simulink model "SCLAING_TRAINING_39"  (R2021a)
settings: Solver=ode23tb  StartTime=0.0  StopTime=27  MaxStep=1/60  RelTol=1e-2  AbsTol=1e-1  EnableMultiTasking=on
PreLoadFcn:
  | NE39bus_data;
  | PSSMODEL=1;
  | LPSS=0;
  | WAPSS=0;
  | WAPSS2=0;
undefined symbols (not defined in the file): AVR_Data, D1, Delta, line, mac_con, MB, Ns, p0, Pn, s
libraries: spsThreePhaseVIMeasurementLib x40, spsThreePhasePISectionLineLib x34, simulink x20, spsGenericPowerSystemStabilizerLib x20, spsThreePhaseTransformerTwoWindingsLib x12, spsSynchronousMachinepuStandardLib x10, spsExcitationSystemLib x10, spsMultiBandPowerSystemStabilizerLib x10, spsSteamTurbineandGovernorLib x10, slpidlib x10, spsLoadFlowBusLib x9, spsThreePhaseDynamicLoadLib x9
(part 4 of 4)

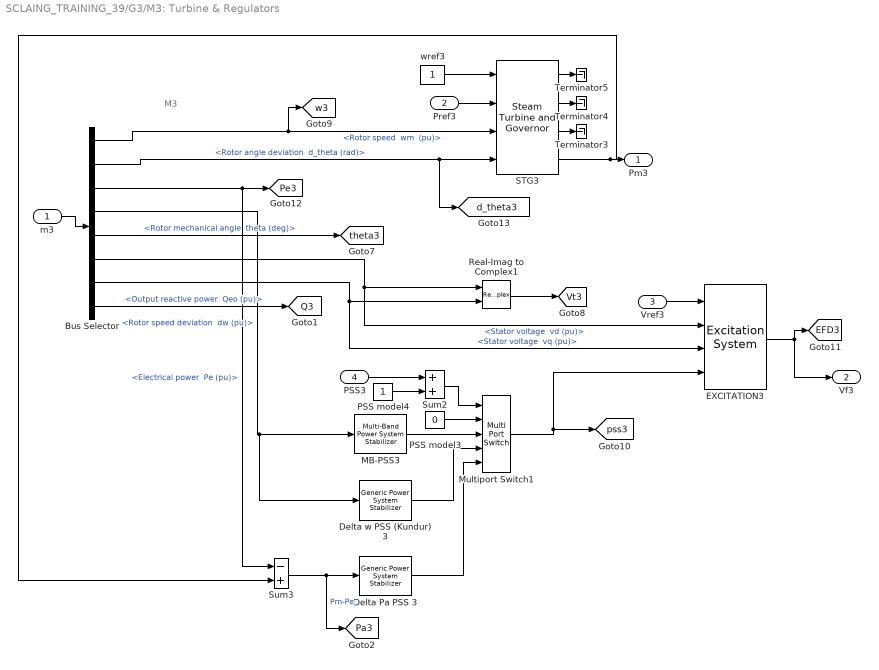
== system SCLAING_TRAINING_39/G3/M3: Turbine & Regulators ==
  note: M3
  m3 : Inport
  Pref3 : Inport  Port=2
  Vref3 : Inport  Port=3
  PSS3 : Inport  Port=4
  Bus Selector : BusSelector  OutputSignals="Mechanical.Rotor speed  wm  (pu),Mechanical.Rotor angle deviation  d_theta (rad),Mechanical.Electrical power  Pe (pu),Mechanical.Rotor speed deviation  dw (pu),Mechanical.Rotor mechanical angle  theta (deg),dq0 components.Stator voltage  vd (pu),dq0 components.Stator voltage  vq (pu),Output reactive power  Qeo (pu)"
  Delta Pa PSS 3 : spsGenericPowerSystemStabilizerLib/Generic Power System Stabilizer  Tsensor=15e-3  K=2.5*1.25  Twashout=1  Tleadlag1=[60e-3 1]  Tleadlag2=[0 0]  VSlimits=[-0.15 0.15]  Vinit=0  Plot_On=off  MagdB_On=on  FreqRange=logspace(-2,2,500)
      settings: SourceProductBaseCode=PS
  Delta w PSS (Kundur) 3 : spsGenericPowerSystemStabilizerLib/Generic Power System Stabilizer  Tsensor=15e-3  K=30  Twashout=10  Tleadlag1=[50e-3 20e-3]  Tleadlag2=[3 5.4]  VSlimits=[-0.15 0.15]  Vinit=0  Plot_On=off  MagdB_On=on  FreqRange=logspace(-2,2,500)
      settings: SourceProductBaseCode=PS
  EXCITATION3 : spsExcitationSystemLib/Excitation System  tr=AVR_Data(3,1)  reg=[ AVR_Data(3,2:3) ]  exc=[ 1, 0 ]  tgr=[ AVR_Data(3,4:5)]  damp=[ 0, 0 ]  sat=[ 0, 0 ]  lim="[ AVR_Data(3,7:8)  0 ]"  v0=[1,2.25944]
      settings: SourceProductBaseCode=PS
  MB-PSS3 : spsMultiBandPowerSystemStabilizerLib/Multi-Band Power System Stabilizer  OperationMode=Simplified settings  Kg=MB(1)  GL=[MB(2) MB(3)]  GI=[MB(4) MB(5)]  GH=[MB(6) MB(7)]  GLd=[66 66 9.4]  TcLF=[1.667 2 0 0 0 0 2 2.4 0 0 0 0 1 1]  GId=[66 66 47.6]  TcIF=[1 1 0.25 0.3 0 0 1 1 0.3 0.36 0 0 0 0]  GHd=[66 66 233]  TcHF="[0.01 0.012 0 0 0 0  0.012 0.0144 0 0 0 0 1 1]"  LIM=[.075 .15 .15 .15]  Plot_On=off  MagdB_On=off  FreqRange=logspace(-2,2,500)
      settings: SourceProductBaseCode=PS
  Multiport Switch1 : MultiPortSwitch  Inputs=4  InputSameDT=on
  PSS model3 : Constant  Value=0
  PSS model4 : Constant
  Real-Imag to Complex1 : RealImagToComplex
  STG3 : spsSteamTurbineandGovernorLib/Steam Turbine and Governor  gentype=Tandem-compound (single mass)  reg1="[ 1  0.05    0 ]"  reg2="[ 0.001  0.15 ]"  reg3="[ -0.1  0.1  0  4.496 ]"  N=Ns  turb1="[ 0  10   3.3   0.5   ]"  turb2="[   0   0.36    0.36   0.28   ]"  HA="[ 0.046  1.430  1.465   0.192 ]"  KA="[ 90.44  53.88  64.59   62.94  ]"  DA="[ 0.0115  0.3575  0.3663   0.0137  ]"  ini1=0.65  ini2=[0.779316,-31.4247]
      settings: SourceProductBaseCode=PS
  Sum2 : Sum  InputSameDT=on  SaturateOnIntegerOverflow=on  OutDataTypeStr=Inherit: Same as first input
  Sum3 : Sum  Inputs=-+  InputSameDT=on  SaturateOnIntegerOverflow=on  OutDataTypeStr=Inherit: Same as first input
  Terminator3 : Terminator
  Terminator4 : Terminator
  Terminator5 : Terminator
  wref3 : Constant
  Pm3 : Outport  InitialOutput=0
  Vf3 : Outport  Port=2  InitialOutput=0
  tag scope: EFD3=global, Pa3=global, Pe3=global, Q3=global, Vt3=global, d_theta3=global, pss3=global, theta3=global, w3=global
  wires:
  Bus Selector/7 -> EXCITATION3/3, Real-Imag to Complex1/2  "<Stator voltage  vq (pu)>"
  wref3/1 -> STG3/1
  Pref3/1 -> STG3/2
  m3/1 -> Bus Selector/1
  Vref3/1 -> EXCITATION3/1
  EXCITATION3/1 -> Vf3/1, [EFD3]
  Real-Imag to Complex1/1 -> [Vt3]
  Bus Selector/5 -> [theta3]  "<Rotor mechanical angle  theta (deg)>"
  Bus Selector/6 -> EXCITATION3/2, Real-Imag to Complex1/1  "<Stator voltage  vd (pu)>"
  STG3/3 -> Terminator3/1
  STG3/4 -> Sum3/2, Pm3/1
  STG3/2 -> Terminator4/1
  STG3/1 -> Terminator5/1
  Bus Selector/1 -> [w3], STG3/3  "<Rotor speed  wm  (pu)>"
  Bus Selector/2 -> STG3/4, [d_theta3]  "<Rotor angle deviation  d_theta (rad)>"
  Bus Selector/3 -> Sum3/1, [Pe3]  "<Electrical power  Pe (pu)>"
  Bus Selector/4 -> Delta w PSS (Kundur) 3/1, MB-PSS3/1  "<Rotor speed deviation  dw (pu)>"
  Bus Selector/8 -> [Q3]  "<Output reactive power  Qeo (pu)>"
  Sum3/1 -> [Pa3], Delta Pa PSS 3/1  "Pm-Pe"
  Sum2/1 -> Multiport Switch1/1
  PSS model4/1 -> Sum2/2
  Delta Pa PSS 3/1 -> Multiport Switch1/5
  Delta w PSS (Kundur) 3/1 -> Multiport Switch1/4
  MB-PSS3/1 -> Multiport Switch1/3
  PSS model3/1 -> Multiport Switch1/2
  Multiport Switch1/1 -> EXCITATION3/4, [pss3]
  PSS3/1 -> Sum2/1

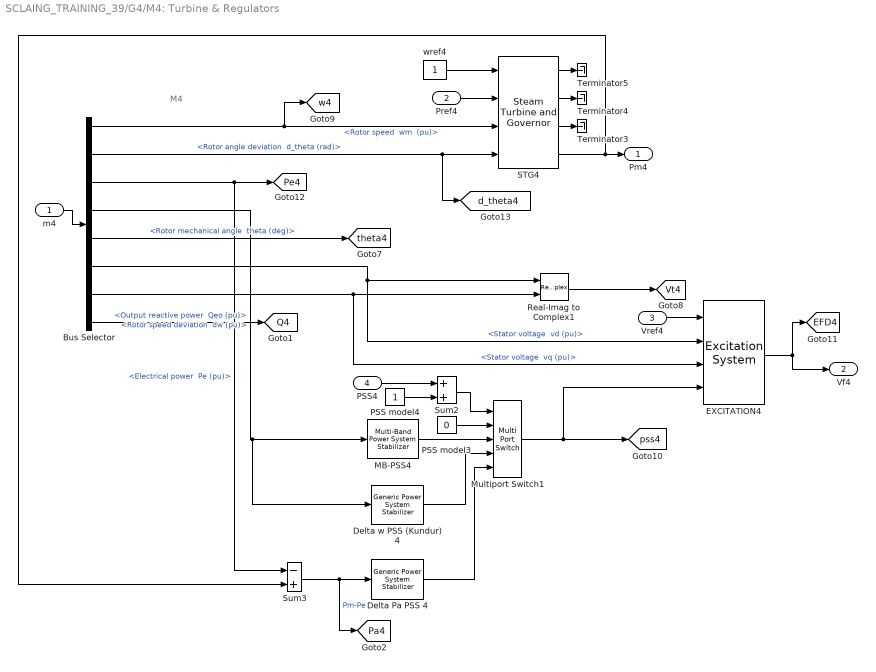
== system SCLAING_TRAINING_39/G4/M4: Turbine & Regulators ==
  note: M4
  m4 : Inport
  Pref4 : Inport  Port=2
  Vref4 : Inport  Port=3
  PSS4 : Inport  Port=4
  Bus Selector : BusSelector  OutputSignals="Mechanical.Rotor speed  wm  (pu),Mechanical.Rotor angle deviation  d_theta (rad),Mechanical.Electrical power  Pe (pu),Mechanical.Rotor speed deviation  dw (pu),Mechanical.Rotor mechanical angle  theta (deg),dq0 components.Stator voltage  vd (pu),dq0 components.Stator voltage  vq (pu),Output reactive power  Qeo (pu)"
  Delta Pa PSS 4 : spsGenericPowerSystemStabilizerLib/Generic Power System Stabilizer  Tsensor=15e-3  K=2.5*1.25  Twashout=1  Tleadlag1=[60e-3 1]  Tleadlag2=[0 0]  VSlimits=[-0.15 0.15]  Vinit=0  Plot_On=off  MagdB_On=on  FreqRange=logspace(-2,2,500)
      settings: SourceProductBaseCode=PS
  Delta w PSS (Kundur) 4 : spsGenericPowerSystemStabilizerLib/Generic Power System Stabilizer  Tsensor=15e-3  K=30  Twashout=10  Tleadlag1=[50e-3 20e-3]  Tleadlag2=[3 5.4]  VSlimits=[-0.15 0.15]  Vinit=0  Plot_On=off  MagdB_On=on  FreqRange=logspace(-2,2,500)
      settings: SourceProductBaseCode=PS
  EXCITATION4 : spsExcitationSystemLib/Excitation System  tr=AVR_Data(1)  reg=[ AVR_Data(4,2:3) ]  exc=[ 1, 0 ]  tgr=[ AVR_Data(4,4:5)]  damp=[ 0, 0 ]  sat=[ 0, 0 ]  lim="[ AVR_Data(4,7:8)  0 ]"  v0=[1,2.14879]
      settings: SourceProductBaseCode=PS
  MB-PSS4 : spsMultiBandPowerSystemStabilizerLib/Multi-Band Power System Stabilizer  OperationMode=Simplified settings  Kg=MB(1)  GL=[MB(2) MB(3)]  GI=[MB(4) MB(5)]  GH=[MB(6) MB(7)]  GLd=[66 66 9.4]  TcLF=[1.667 2 0 0 0 0 2 2.4 0 0 0 0 1 1]  GId=[66 66 47.6]  TcIF=[1 1 0.25 0.3 0 0 1 1 0.3 0.36 0 0 0 0]  GHd=[66 66 233]  TcHF="[0.01 0.012 0 0 0 0  0.012 0.0144 0 0 0 0 1 1]"  LIM=[.075 .15 .15 .15]  Plot_On=off  MagdB_On=off  FreqRange=logspace(-2,2,500)
      settings: SourceProductBaseCode=PS
  Multiport Switch1 : MultiPortSwitch  Inputs=4  InputSameDT=on
  PSS model3 : Constant  Value=0
  PSS model4 : Constant
  Real-Imag to Complex1 : RealImagToComplex
  STG4 : spsSteamTurbineandGovernorLib/Steam Turbine and Governor  gentype=Tandem-compound (single mass)  reg1="[ 1  0.05    0 ]"  reg2="[ 0.001  0.15 ]"  reg3="[ -0.1  0.1  0  4.496 ]"  N=Ns  turb1="[ 0  10   3.3   0.5   ]"  turb2="[   0   0.36    0.36   0.28   ]"  HA="[ 0.046  1.430  1.465   0.192 ]"  KA="[ 90.44  53.88  64.59   62.94  ]"  DA="[ 0.0115  0.3575  0.3663   0.0137  ]"  ini1=0.632  ini2=[0.779316,-31.4247]
      settings: SourceProductBaseCode=PS
  Sum2 : Sum  InputSameDT=on  SaturateOnIntegerOverflow=on  OutDataTypeStr=Inherit: Same as first input
  Sum3 : Sum  Inputs=-+  InputSameDT=on  SaturateOnIntegerOverflow=on  OutDataTypeStr=Inherit: Same as first input
  Terminator3 : Terminator
  Terminator4 : Terminator
  Terminator5 : Terminator
  wref4 : Constant
  Pm4 : Outport  InitialOutput=0
  Vf4 : Outport  Port=2  InitialOutput=0
  tag scope: EFD4=global, Pa4=global, Pe4=global, Q4=global, Vt4=global, d_theta4=global, pss4=global, theta4=global, w4=global
  wires:
  Bus Selector/7 -> EXCITATION4/3, Real-Imag to Complex1/2  "<Stator voltage  vq (pu)>"
  wref4/1 -> STG4/1
  Pref4/1 -> STG4/2
  m4/1 -> Bus Selector/1
  Vref4/1 -> EXCITATION4/1
  EXCITATION4/1 -> Vf4/1, [EFD4]
  Real-Imag to Complex1/1 -> [Vt4]
  Bus Selector/5 -> [theta4]  "<Rotor mechanical angle  theta (deg)>"
  Bus Selector/6 -> EXCITATION4/2, Real-Imag to Complex1/1  "<Stator voltage  vd (pu)>"
  STG4/3 -> Terminator3/1
  STG4/4 -> Sum3/2, Pm4/1
  STG4/2 -> Terminator4/1
  STG4/1 -> Terminator5/1
  Bus Selector/1 -> [w4], STG4/3  "<Rotor speed  wm  (pu)>"
  Bus Selector/2 -> [d_theta4], STG4/4  "<Rotor angle deviation  d_theta (rad)>"
  Bus Selector/3 -> Sum3/1, [Pe4]  "<Electrical power  Pe (pu)>"
  Bus Selector/4 -> Delta w PSS (Kundur) 4/1, MB-PSS4/1  "<Rotor speed deviation  dw (pu)>"
  Bus Selector/8 -> [Q4]  "<Output reactive power  Qeo (pu)>"
  Sum3/1 -> [Pa4], Delta Pa PSS 4/1  "Pm-Pe"
  Sum2/1 -> Multiport Switch1/1
  PSS model4/1 -> Sum2/2
  Delta Pa PSS 4/1 -> Multiport Switch1/5
  Delta w PSS (Kundur) 4/1 -> Multiport Switch1/4
  MB-PSS4/1 -> Multiport Switch1/3
  PSS model3/1 -> Multiport Switch1/2
  Multiport Switch1/1 -> [pss4], EXCITATION4/4
  PSS4/1 -> Sum2/1

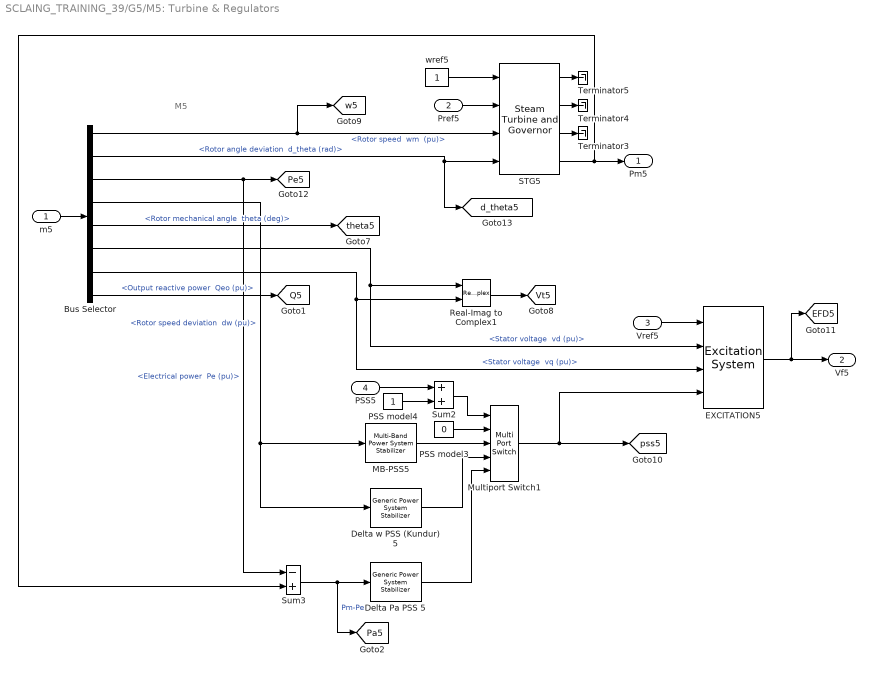
== system SCLAING_TRAINING_39/G5/M5: Turbine & Regulators ==
  note: M5
  m5 : Inport
  Pref5 : Inport  Port=2
  Vref5 : Inport  Port=3
  PSS5 : Inport  Port=4
  Bus Selector : BusSelector  OutputSignals="Mechanical.Rotor speed  wm  (pu),Mechanical.Rotor angle deviation  d_theta (rad),Mechanical.Electrical power  Pe (pu),Mechanical.Rotor speed deviation  dw (pu),Mechanical.Rotor mechanical angle  theta (deg),dq0 components.Stator voltage  vd (pu),dq0 components.Stator voltage  vq (pu),Output reactive power  Qeo (pu)"
  Delta Pa PSS 5 : spsGenericPowerSystemStabilizerLib/Generic Power System Stabilizer  Tsensor=15e-3  K=2.5*1.25  Twashout=1  Tleadlag1=[60e-3 1]  Tleadlag2=[0 0]  VSlimits=[-0.15 0.15]  Vinit=0  Plot_On=off  MagdB_On=on  FreqRange=logspace(-2,2,500)
      settings: SourceProductBaseCode=PS
  Delta w PSS (Kundur) 5 : spsGenericPowerSystemStabilizerLib/Generic Power System Stabilizer  Tsensor=15e-3  K=30  Twashout=10  Tleadlag1=[50e-3 20e-3]  Tleadlag2=[3 5.4]  VSlimits=[-0.15 0.15]  Vinit=0  Plot_On=off  MagdB_On=on  FreqRange=logspace(-2,2,500)
      settings: SourceProductBaseCode=PS
  EXCITATION5 : spsExcitationSystemLib/Excitation System  tr=AVR_Data(5,1)  reg=[ AVR_Data(5,2:3) ]  exc=[ 1, 0 ]  tgr=[ AVR_Data(5,4:5)]  damp=[ 0, 0 ]  sat=[ 0, 0 ]  lim="[ AVR_Data(5,7:8)  0 ]"  v0=[1,3.89055]
      settings: SourceProductBaseCode=PS
  MB-PSS5 : spsMultiBandPowerSystemStabilizerLib/Multi-Band Power System Stabilizer  OperationMode=Simplified settings  Kg=MB(1)  GL=[MB(2) MB(3)]  GI=[MB(4) MB(5)]  GH=[MB(6) MB(7)]  GLd=[66 66 9.4]  TcLF=[1.667 2 0 0 0 0 2 2.4 0 0 0 0 1 1]  GId=[66 66 47.6]  TcIF=[1 1 0.25 0.3 0 0 1 1 0.3 0.36 0 0 0 0]  GHd=[66 66 233]  TcHF="[0.01 0.012 0 0 0 0  0.012 0.0144 0 0 0 0 1 1]"  LIM=[.075 .15 .15 .15]  Plot_On=off  MagdB_On=off  FreqRange=logspace(-2,2,500)
      settings: SourceProductBaseCode=PS
  Multiport Switch1 : MultiPortSwitch  Inputs=4  InputSameDT=on
  PSS model3 : Constant  Value=0
  PSS model4 : Constant
  Real-Imag to Complex1 : RealImagToComplex
  STG5 : spsSteamTurbineandGovernorLib/Steam Turbine and Governor  gentype=Tandem-compound (single mass)  reg1="[ 1  0.05    0 ]"  reg2="[ 0.001  0.15 ]"  reg3="[ -0.1  0.1  0  4.496 ]"  N=Ns  turb1="[ 0  10   3.3   0.5   ]"  turb2="[   0   0.36    0.36   0.28   ]"  HA="[ 0.046  1.430  1.465   0.192 ]"  KA="[ 90.44  53.88  64.59   62.94  ]"  DA="[ 0.0115  0.3575  0.3663   0.0137  ]"  ini1=0.508  ini2=[0.779316,-31.4247]
      settings: SourceProductBaseCode=PS
  Sum2 : Sum  InputSameDT=on  SaturateOnIntegerOverflow=on  OutDataTypeStr=Inherit: Same as first input
  Sum3 : Sum  Inputs=-+  InputSameDT=on  SaturateOnIntegerOverflow=on  OutDataTypeStr=Inherit: Same as first input
  Terminator3 : Terminator
  Terminator4 : Terminator
  Terminator5 : Terminator
  wref5 : Constant
  Pm5 : Outport  InitialOutput=0
  Vf5 : Outport  Port=2  InitialOutput=0
  tag scope: EFD5=global, Pa5=global, Pe5=global, Q5=global, Vt5=global, d_theta5=global, pss5=global, theta5=global, w5=global
  wires:
  Bus Selector/7 -> EXCITATION5/3, Real-Imag to Complex1/2  "<Stator voltage  vq (pu)>"
  wref5/1 -> STG5/1
  Pref5/1 -> STG5/2
  m5/1 -> Bus Selector/1
  Vref5/1 -> EXCITATION5/1
  EXCITATION5/1 -> Vf5/1, [EFD5]
  Real-Imag to Complex1/1 -> [Vt5]
  Bus Selector/5 -> [theta5]  "<Rotor mechanical angle  theta (deg)>"
  Bus Selector/6 -> EXCITATION5/2, Real-Imag to Complex1/1  "<Stator voltage  vd (pu)>"
  STG5/3 -> Terminator3/1
  STG5/4 -> Sum3/2, Pm5/1
  STG5/2 -> Terminator4/1
  STG5/1 -> Terminator5/1
  Bus Selector/1 -> [w5], STG5/3  "<Rotor speed  wm  (pu)>"
  Bus Selector/2 -> [d_theta5], STG5/4  "<Rotor angle deviation  d_theta (rad)>"
  Bus Selector/3 -> Sum3/1, [Pe5]  "<Electrical power  Pe (pu)>"
  Bus Selector/4 -> Delta w PSS (Kundur) 5/1, MB-PSS5/1  "<Rotor speed deviation  dw (pu)>"
  Bus Selector/8 -> [Q5]  "<Output reactive power  Qeo (pu)>"
  Sum3/1 -> [Pa5], Delta Pa PSS 5/1  "Pm-Pe"
  Sum2/1 -> Multiport Switch1/1
  PSS model4/1 -> Sum2/2
  Delta Pa PSS 5/1 -> Multiport Switch1/5
  Delta w PSS (Kundur) 5/1 -> Multiport Switch1/4
  MB-PSS5/1 -> Multiport Switch1/3
  PSS model3/1 -> Multiport Switch1/2
  Multiport Switch1/1 -> [pss5], EXCITATION5/4
  PSS5/1 -> Sum2/1

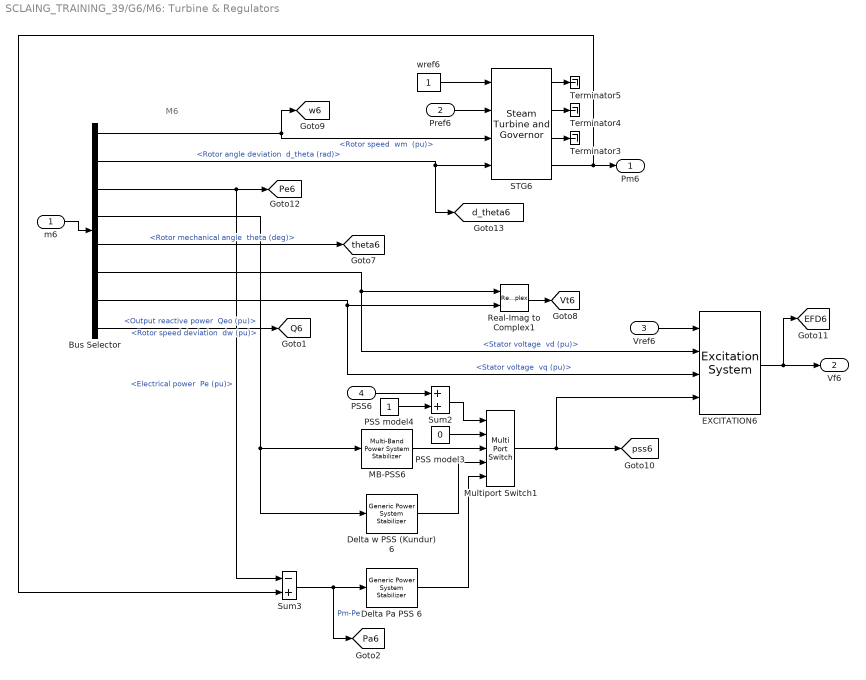
== system SCLAING_TRAINING_39/G6/M6: Turbine & Regulators ==
  note: M6
  m6 : Inport
  Pref6 : Inport  Port=2
  Vref6 : Inport  Port=3
  PSS6 : Inport  Port=4
  Bus Selector : BusSelector  OutputSignals="Mechanical.Rotor speed  wm  (pu),Mechanical.Rotor angle deviation  d_theta (rad),Mechanical.Electrical power  Pe (pu),Mechanical.Rotor speed deviation  dw (pu),Mechanical.Rotor mechanical angle  theta (deg),dq0 components.Stator voltage  vd (pu),dq0 components.Stator voltage  vq (pu),Output reactive power  Qeo (pu)"
  Delta Pa PSS 6 : spsGenericPowerSystemStabilizerLib/Generic Power System Stabilizer  Tsensor=15e-3  K=2.5*1.25  Twashout=1  Tleadlag1=[60e-3 1]  Tleadlag2=[0 0]  VSlimits=[-0.15 0.15]  Vinit=0  Plot_On=off  MagdB_On=on  FreqRange=logspace(-2,2,500)
      settings: SourceProductBaseCode=PS
  Delta w PSS (Kundur) 6 : spsGenericPowerSystemStabilizerLib/Generic Power System Stabilizer  Tsensor=15e-3  K=30  Twashout=10  Tleadlag1=[50e-3 20e-3]  Tleadlag2=[3 5.4]  VSlimits=[-0.15 0.15]  Vinit=0  Plot_On=off  MagdB_On=on  FreqRange=logspace(-2,2,500)
      settings: SourceProductBaseCode=PS
  EXCITATION6 : spsExcitationSystemLib/Excitation System  tr=AVR_Data(6,1)  reg=[ AVR_Data(6,2:3) ]  exc=[ 1, 0 ]  tgr=[ AVR_Data(6,4:5)]  damp=[ 0, 0 ]  sat=[ 0, 0 ]  lim="[ AVR_Data(6,7:8)  0 ]"  v0=[1,2.21937]
      settings: SourceProductBaseCode=PS
  MB-PSS6 : spsMultiBandPowerSystemStabilizerLib/Multi-Band Power System Stabilizer  OperationMode=Simplified settings  Kg=MB(1)  GL=[MB(2) MB(3)]  GI=[MB(4) MB(5)]  GH=[MB(6) MB(7)]  GLd=[66 66 9.4]  TcLF=[1.667 2 0 0 0 0 2 2.4 0 0 0 0 1 1]  GId=[66 66 47.6]  TcIF=[1 1 0.25 0.3 0 0 1 1 0.3 0.36 0 0 0 0]  GHd=[66 66 233]  TcHF="[0.01 0.012 0 0 0 0  0.012 0.0144 0 0 0 0 1 1]"  LIM=[.075 .15 .15 .15]  Plot_On=off  MagdB_On=off  FreqRange=logspace(-2,2,500)
      settings: SourceProductBaseCode=PS
  Multiport Switch1 : MultiPortSwitch  Inputs=4  InputSameDT=on
  PSS model3 : Constant  Value=0
  PSS model4 : Constant
  Real-Imag to Complex1 : RealImagToComplex
  STG6 : spsSteamTurbineandGovernorLib/Steam Turbine and Governor  gentype=Tandem-compound (single mass)  reg1="[ 1  0.05    0 ]"  reg2="[ 0.001  0.15 ]"  reg3="[ -0.1  0.1  0  4.496 ]"  N=Ns  turb1="[ 0  10   3.3   0.5   ]"  turb2="[   0   0.36    0.36   0.28   ]"  HA="[ 0.046  1.430  1.465   0.192 ]"  KA="[ 90.44  53.88  64.59   62.94  ]"  DA="[ 0.0115  0.3575  0.3663   0.0137  ]"  ini1=0.65  ini2=[0.779316,-31.4247]
      settings: SourceProductBaseCode=PS
  Sum2 : Sum  InputSameDT=on  SaturateOnIntegerOverflow=on  OutDataTypeStr=Inherit: Same as first input
  Sum3 : Sum  Inputs=-+  InputSameDT=on  SaturateOnIntegerOverflow=on  OutDataTypeStr=Inherit: Same as first input
  Terminator3 : Terminator
  Terminator4 : Terminator
  Terminator5 : Terminator
  wref6 : Constant
  Pm6 : Outport  InitialOutput=0
  Vf6 : Outport  Port=2  InitialOutput=0
  tag scope: EFD6=global, Pa6=global, Pe6=global, Q6=global, Vt6=global, d_theta6=global, pss6=global, theta6=global, w6=global
  wires:
  Bus Selector/7 -> EXCITATION6/3, Real-Imag to Complex1/2  "<Stator voltage  vq (pu)>"
  wref6/1 -> STG6/1
  Pref6/1 -> STG6/2
  m6/1 -> Bus Selector/1
  Vref6/1 -> EXCITATION6/1
  EXCITATION6/1 -> Vf6/1, [EFD6]
  Real-Imag to Complex1/1 -> [Vt6]
  Bus Selector/5 -> [theta6]  "<Rotor mechanical angle  theta (deg)>"
  Bus Selector/6 -> EXCITATION6/2, Real-Imag to Complex1/1  "<Stator voltage  vd (pu)>"
  STG6/3 -> Terminator3/1
  STG6/4 -> Sum3/2, Pm6/1
  STG6/2 -> Terminator4/1
  STG6/1 -> Terminator5/1
  Bus Selector/1 -> STG6/3, [w6]  "<Rotor speed  wm  (pu)>"
  Bus Selector/2 -> [d_theta6], STG6/4  "<Rotor angle deviation  d_theta (rad)>"
  Bus Selector/3 -> Sum3/1, [Pe6]  "<Electrical power  Pe (pu)>"
  Bus Selector/4 -> Delta w PSS (Kundur) 6/1, MB-PSS6/1  "<Rotor speed deviation  dw (pu)>"
  Bus Selector/8 -> [Q6]  "<Output reactive power  Qeo (pu)>"
  Sum3/1 -> [Pa6], Delta Pa PSS 6/1  "Pm-Pe"
  Sum2/1 -> Multiport Switch1/1
  PSS model4/1 -> Sum2/2
  Delta Pa PSS 6/1 -> Multiport Switch1/5
  Delta w PSS (Kundur) 6/1 -> Multiport Switch1/4
  MB-PSS6/1 -> Multiport Switch1/3
  PSS model3/1 -> Multiport Switch1/2
  Multiport Switch1/1 -> [pss6], EXCITATION6/4
  PSS6/1 -> Sum2/1

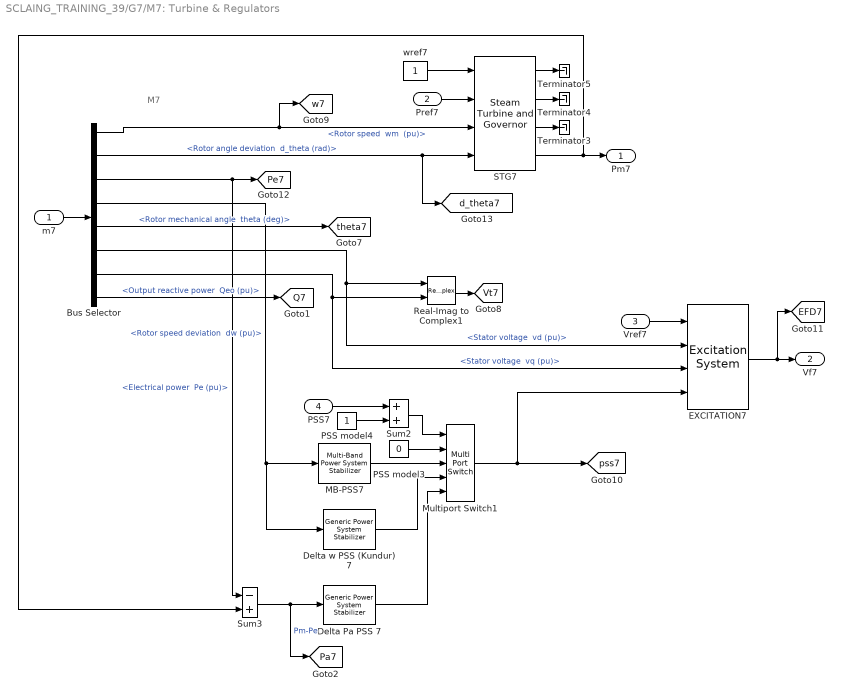
== system SCLAING_TRAINING_39/G7/M7: Turbine & Regulators ==
  note: M7
  m7 : Inport
  Pref7 : Inport  Port=2
  Vref7 : Inport  Port=3
  PSS7 : Inport  Port=4
  Bus Selector : BusSelector  OutputSignals="Mechanical.Rotor speed  wm  (pu),Mechanical.Rotor angle deviation  d_theta (rad),Mechanical.Electrical power  Pe (pu),Mechanical.Rotor speed deviation  dw (pu),Mechanical.Rotor mechanical angle  theta (deg),dq0 components.Stator voltage  vd (pu),dq0 components.Stator voltage  vq (pu),Output reactive power  Qeo (pu)"
  Delta Pa PSS 7 : spsGenericPowerSystemStabilizerLib/Generic Power System Stabilizer  Tsensor=15e-3  K=2.5*1.25  Twashout=1  Tleadlag1=[60e-3 1]  Tleadlag2=[0 0]  VSlimits=[-0.15 0.15]  Vinit=0  Plot_On=off  MagdB_On=on  FreqRange=logspace(-2,2,500)
      settings: SourceProductBaseCode=PS
  Delta w PSS (Kundur) 7 : spsGenericPowerSystemStabilizerLib/Generic Power System Stabilizer  Tsensor=15e-3  K=30  Twashout=10  Tleadlag1=[50e-3 20e-3]  Tleadlag2=[3 5.4]  VSlimits=[-0.15 0.15]  Vinit=0  Plot_On=off  MagdB_On=on  FreqRange=logspace(-2,2,500)
      settings: SourceProductBaseCode=PS
  EXCITATION7 : spsExcitationSystemLib/Excitation System  tr=AVR_Data(7,1)  reg=[ AVR_Data(7,2:3) ]  exc=[ 1, 0 ]  tgr=[ AVR_Data(7,4:5)]  damp=[ 0, 0 ]  sat=[ 0, 0 ]  lim="[ AVR_Data(7,7:8)  0 ]"  v0=[1,2.15543]
      settings: SourceProductBaseCode=PS
  MB-PSS7 : spsMultiBandPowerSystemStabilizerLib/Multi-Band Power System Stabilizer  OperationMode=Simplified settings  Kg=MB(1)  GL=[MB(2) MB(3)]  GI=[MB(4) MB(5)]  GH=[MB(6) MB(7)]  GLd=[66 66 9.4]  TcLF=[1.667 2 0 0 0 0 2 2.4 0 0 0 0 1 1]  GId=[66 66 47.6]  TcIF=[1 1 0.25 0.3 0 0 1 1 0.3 0.36 0 0 0 0]  GHd=[66 66 233]  TcHF="[0.01 0.012 0 0 0 0  0.012 0.0144 0 0 0 0 1 1]"  LIM=[.075 .15 .15 .15]  Plot_On=off  MagdB_On=off  FreqRange=logspace(-2,2,500)
      settings: SourceProductBaseCode=PS
  Multiport Switch1 : MultiPortSwitch  Inputs=4  InputSameDT=on
  PSS model3 : Constant  Value=0
  PSS model4 : Constant
  Real-Imag to Complex1 : RealImagToComplex
  STG7 : spsSteamTurbineandGovernorLib/Steam Turbine and Governor  gentype=Tandem-compound (single mass)  reg1="[ 1  0.05    0 ]"  reg2="[ 0.001  0.15 ]"  reg3="[ -0.1  0.1  0  4.496 ]"  N=Ns  turb1="[ 0  10   3.3   0.5   ]"  turb2="[   0   0.36    0.36   0.28   ]"  HA="[ 0.046  1.430  1.465   0.192 ]"  KA="[ 90.44  53.88  64.59   62.94  ]"  DA="[ 0.0115  0.3575  0.3663   0.0137  ]"  ini1=0.56  ini2=[0.779316,-31.4247]
      settings: SourceProductBaseCode=PS
  Sum2 : Sum  InputSameDT=on  SaturateOnIntegerOverflow=on  OutDataTypeStr=Inherit: Same as first input
  Sum3 : Sum  Inputs=-+  InputSameDT=on  SaturateOnIntegerOverflow=on  OutDataTypeStr=Inherit: Same as first input
  Terminator3 : Terminator
  Terminator4 : Terminator
  Terminator5 : Terminator
  wref7 : Constant
  Pm7 : Outport  InitialOutput=0
  Vf7 : Outport  Port=2  InitialOutput=0
  tag scope: EFD7=global, Pa7=global, Pe7=global, Q7=global, Vt7=global, d_theta7=global, pss7=global, theta7=global, w7=global
  wires:
  Bus Selector/7 -> EXCITATION7/3, Real-Imag to Complex1/2  "<Stator voltage  vq (pu)>"
  wref7/1 -> STG7/1
  Pref7/1 -> STG7/2
  m7/1 -> Bus Selector/1
  Vref7/1 -> EXCITATION7/1
  EXCITATION7/1 -> Vf7/1, [EFD7]
  Real-Imag to Complex1/1 -> [Vt7]
  Bus Selector/5 -> [theta7]  "<Rotor mechanical angle  theta (deg)>"
  Bus Selector/6 -> EXCITATION7/2, Real-Imag to Complex1/1  "<Stator voltage  vd (pu)>"
  STG7/3 -> Terminator3/1
  STG7/4 -> Sum3/2, Pm7/1
  STG7/2 -> Terminator4/1
  STG7/1 -> Terminator5/1
  Bus Selector/1 -> [w7], STG7/3  "<Rotor speed  wm  (pu)>"
  Bus Selector/2 -> STG7/4, [d_theta7]  "<Rotor angle deviation  d_theta (rad)>"
  Bus Selector/3 -> Sum3/1, [Pe7]  "<Electrical power  Pe (pu)>"
  Bus Selector/4 -> Delta w PSS (Kundur) 7/1, MB-PSS7/1  "<Rotor speed deviation  dw (pu)>"
  Bus Selector/8 -> [Q7]  "<Output reactive power  Qeo (pu)>"
  Sum3/1 -> [Pa7], Delta Pa PSS 7/1  "Pm-Pe"
  Sum2/1 -> Multiport Switch1/1
  PSS model4/1 -> Sum2/2
  Delta Pa PSS 7/1 -> Multiport Switch1/5
  Delta w PSS (Kundur) 7/1 -> Multiport Switch1/4
  MB-PSS7/1 -> Multiport Switch1/3
  PSS model3/1 -> Multiport Switch1/2
  Multiport Switch1/1 -> EXCITATION7/4, [pss7]
  PSS7/1 -> Sum2/1

== system SCLAING_TRAINING_39/G8/M8: Turbine & Regulators ==
  note: M8
  m8 : Inport
  Pref8 : Inport  Port=2
  Vref8 : Inport  Port=3
  PSS8 : Inport  Port=4
  Bus Selector : BusSelector  OutputSignals="Mechanical.Rotor speed  wm  (pu),Mechanical.Rotor angle deviation  d_theta (rad),Mechanical.Electrical power  Pe (pu),Mechanical.Rotor speed deviation  dw (pu),Mechanical.Rotor mechanical angle  theta (deg),dq0 components.Stator voltage  vd (pu),dq0 components.Stator voltage  vq (pu),Output reactive power  Qeo (pu)"
  Delta Pa PSS 8 : spsGenericPowerSystemStabilizerLib/Generic Power System Stabilizer  Tsensor=15e-3  K=2.5*1.25  Twashout=1  Tleadlag1=[60e-3 1]  Tleadlag2=[0 0]  VSlimits=[-0.15 0.15]  Vinit=0  Plot_On=off  MagdB_On=on  FreqRange=logspace(-2,2,500)
      settings: SourceProductBaseCode=PS
  Delta w PSS (Kundur) 8 : spsGenericPowerSystemStabilizerLib/Generic Power System Stabilizer  Tsensor=15e-3  K=30  Twashout=10  Tleadlag1=[50e-3 20e-3]  Tleadlag2=[3 5.4]  VSlimits=[-0.15 0.15]  Vinit=0  Plot_On=off  MagdB_On=on  FreqRange=logspace(-2,2,500)
      settings: SourceProductBaseCode=PS
  EXCITATION8 : spsExcitationSystemLib/Excitation System  tr=AVR_Data(8,1)  reg=[ AVR_Data(8,2:3) ]  exc=[ 1, 0 ]  tgr=[ AVR_Data(8,4:5)]  damp=[ 0, 0 ]  sat=[ 0, 0 ]  lim="[ AVR_Data(8,7:8)  0 ]"  v0=[1,1.90805]
      settings: SourceProductBaseCode=PS
  MB-PSS8 : spsMultiBandPowerSystemStabilizerLib/Multi-Band Power System Stabilizer  OperationMode=Simplified settings  Kg=MB(1)  GL=[MB(2) MB(3)]  GI=[MB(4) MB(5)]  GH=[MB(6) MB(7)]  GLd=[66 66 9.4]  TcLF=[1.667 2 0 0 0 0 2 2.4 0 0 0 0 1 1]  GId=[66 66 47.6]  TcIF=[1 1 0.25 0.3 0 0 1 1 0.3 0.36 0 0 0 0]  GHd=[66 66 233]  TcHF="[0.01 0.012 0 0 0 0  0.012 0.0144 0 0 0 0 1 1]"  LIM=[.075 .15 .15 .15]  Plot_On=off  MagdB_On=off  FreqRange=logspace(-2,2,500)
      settings: SourceProductBaseCode=PS
  Multiport Switch2 : MultiPortSwitch  Inputs=4  InputSameDT=on
  PSS model1 : Constant  Value=0
  PSS model2 : Constant
  Real-Imag to Complex1 : RealImagToComplex
  STG8 : spsSteamTurbineandGovernorLib/Steam Turbine and Governor  gentype=Tandem-compound (single mass)  reg1="[ 1  0.05    0 ]"  reg2="[ 0.001  0.15 ]"  reg3="[ -0.1  0.1  0  4.496 ]"  N=Ns  turb1="[ 0  10   3.3   0.5   ]"  turb2="[   0   0.36    0.36   0.28   ]"  HA="[ 0.046  1.430  1.465   0.192 ]"  KA="[ 90.44  53.88  64.59   62.94  ]"  DA="[ 0.0115  0.3575  0.3663   0.0137  ]"  ini1=0.54  ini2=[0.779316,-31.4247]
      settings: SourceProductBaseCode=PS
  Sum1 : Sum  Inputs=-+  InputSameDT=on  SaturateOnIntegerOverflow=on  OutDataTypeStr=Inherit: Same as first input
  Sum2 : Sum  InputSameDT=on  SaturateOnIntegerOverflow=on  OutDataTypeStr=Inherit: Same as first input
  Terminator3 : Terminator
  Terminator4 : Terminator
  Terminator5 : Terminator
  wref8 : Constant
  Pm8 : Outport  InitialOutput=0
  Vf8 : Outport  Port=2  InitialOutput=0
  tag scope: EFD8=global, Pa8=global, Pe8=global, Q8=global, Vt8=global, d_theta8=global, pss8=global, theta8=global, w8=global
  wires:
  Bus Selector/7 -> EXCITATION8/3, Real-Imag to Complex1/2  "<Stator voltage  vq (pu)>"
  wref8/1 -> STG8/1
  Pref8/1 -> STG8/2
  m8/1 -> Bus Selector/1
  Vref8/1 -> EXCITATION8/1
  EXCITATION8/1 -> Vf8/1, [EFD8]
  Real-Imag to Complex1/1 -> [Vt8]
  Bus Selector/5 -> [theta8]  "<Rotor mechanical angle  theta (deg)>"
  Bus Selector/6 -> EXCITATION8/2, Real-Imag to Complex1/1  "<Stator voltage  vd (pu)>"
  STG8/3 -> Terminator3/1
  STG8/4 -> Sum1/2, Pm8/1
  STG8/2 -> Terminator4/1
  STG8/1 -> Terminator5/1
  Bus Selector/1 -> [w8], STG8/3  "<Rotor speed  wm  (pu)>"
  Bus Selector/2 -> STG8/4, [d_theta8]  "<Rotor angle deviation  d_theta (rad)>"
  Bus Selector/3 -> Sum1/1, [Pe8]  "<Electrical power  Pe (pu)>"
  Bus Selector/4 -> MB-PSS8/1, Delta w PSS (Kundur) 8/1  "<Rotor speed deviation  dw (pu)>"
  Bus Selector/8 -> [Q8]  "<Output reactive power  Qeo (pu)>"
  Sum1/1 -> [Pa8], Delta Pa PSS 8/1  "Pm-Pe"
  Sum2/1 -> Multiport Switch2/1
  PSS model2/1 -> Sum2/2
  Delta Pa PSS 8/1 -> Multiport Switch2/5
  Delta w PSS (Kundur) 8/1 -> Multiport Switch2/4
  MB-PSS8/1 -> Multiport Switch2/3
  PSS model1/1 -> Multiport Switch2/2
  Multiport Switch2/1 -> EXCITATION8/4, [pss8]
  PSS8/1 -> Sum2/1

== system SCLAING_TRAINING_39/G9/M9: Turbine & Regulators  ==
  note: M9
  m9 : Inport
  Pref9 : Inport  Port=2
  Vref9 : Inport  Port=3
  PSS9 : Inport  Port=4
  Bus Selector : BusSelector  OutputSignals="Mechanical.Rotor speed  wm  (pu),Mechanical.Rotor angle deviation  d_theta (rad),Mechanical.Electrical power  Pe (pu),Mechanical.Rotor speed deviation  dw (pu),Mechanical.Rotor mechanical angle  theta (deg),dq0 components.Stator voltage  vd (pu),dq0 components.Stator voltage  vq (pu),Output reactive power  Qeo (pu)"
  Delta Pa PSS 9 : spsGenericPowerSystemStabilizerLib/Generic Power System Stabilizer  Tsensor=15e-3  K=2.5*1.25  Twashout=1  Tleadlag1=[60e-3 1]  Tleadlag2=[0 0]  VSlimits=[-0.15 0.15]  Vinit=0  Plot_On=off  MagdB_On=on  FreqRange=logspace(-2,2,500)
      settings: SourceProductBaseCode=PS
  Delta w PSS (Kundur) 9 : spsGenericPowerSystemStabilizerLib/Generic Power System Stabilizer  Tsensor=15e-3  K=30  Twashout=10  Tleadlag1=[50e-3 20e-3]  Tleadlag2=[3 5.4]  VSlimits=[-0.15 0.15]  Vinit=0  Plot_On=off  MagdB_On=on  FreqRange=logspace(-2,2,500)
      settings: SourceProductBaseCode=PS
  EXCITATION9 : spsExcitationSystemLib/Excitation System  tr=AVR_Data(9,1)  reg=[ AVR_Data(9,2:3) ]  exc=[ 1, 0 ]  tgr=[ AVR_Data(9,4:5)]  damp=[ 0, 0 ]  sat=[ 0, 0 ]  lim="[ AVR_Data(9,7:8)  0 ]"  v0=[1,2.08155]
      settings: SourceProductBaseCode=PS
  MB-PSS9 : spsMultiBandPowerSystemStabilizerLib/Multi-Band Power System Stabilizer  OperationMode=Simplified settings  Kg=MB(1)  GL=[MB(2) MB(3)]  GI=[MB(4) MB(5)]  GH=[MB(6) MB(7)]  GLd=[66 66 9.4]  TcLF=[1.667 2 0 0 0 0 2 2.4 0 0 0 0 1 1]  GId=[66 66 47.6]  TcIF=[1 1 0.25 0.3 0 0 1 1 0.3 0.36 0 0 0 0]  GHd=[66 66 233]  TcHF="[0.01 0.012 0 0 0 0  0.012 0.0144 0 0 0 0 1 1]"  LIM=[.075 .15 .15 .15]  Plot_On=off  MagdB_On=off  FreqRange=logspace(-2,2,500)
      settings: SourceProductBaseCode=PS
  Multiport Switch1 : MultiPortSwitch  Inputs=4  InputSameDT=on
  PSS model3 : Constant  Value=0
  PSS model4 : Constant
  Real-Imag to Complex1 : RealImagToComplex
  STG9 : spsSteamTurbineandGovernorLib/Steam Turbine and Governor  gentype=Tandem-compound (single mass)  reg1="[ 1  0.05    0 ]"  reg2="[ 0.001  0.15 ]"  reg3="[ -0.1  0.1  0  4.496 ]"  N=Ns  turb1="[ 0  10   3.3   0.5   ]"  turb2="[   0   0.36    0.36   0.28   ]"  HA="[ 0.046  1.430  1.465   0.192 ]"  KA="[ 90.44  53.88  64.59   62.94  ]"  DA="[ 0.0115  0.3575  0.3663   0.0137  ]"  ini1=0.83  ini2=[0.779316,-31.4247]
      settings: SourceProductBaseCode=PS
  Sum2 : Sum  InputSameDT=on  SaturateOnIntegerOverflow=on  OutDataTypeStr=Inherit: Same as first input
  Sum3 : Sum  Inputs=-+  InputSameDT=on  SaturateOnIntegerOverflow=on  OutDataTypeStr=Inherit: Same as first input
  Terminator3 : Terminator
  Terminator4 : Terminator
  Terminator5 : Terminator
  wref9 : Constant
  Pm9 : Outport  InitialOutput=0
  Vf9 : Outport  Port=2  InitialOutput=0
  tag scope: EFD9=global, Pa9=global, Pe9=global, Q9=global, Vt9=global, d_theta9=global, pss9=global, theta9=global, w9=global
  wires:
  Bus Selector/7 -> EXCITATION9/3, Real-Imag to Complex1/2  "<Stator voltage  vq (pu)>"
  wref9/1 -> STG9/1
  Pref9/1 -> STG9/2
  m9/1 -> Bus Selector/1
  Vref9/1 -> EXCITATION9/1
  EXCITATION9/1 -> Vf9/1, [EFD9]
  Real-Imag to Complex1/1 -> [Vt9]
  Bus Selector/5 -> [theta9]  "<Rotor mechanical angle  theta (deg)>"
  Bus Selector/6 -> EXCITATION9/2, Real-Imag to Complex1/1  "<Stator voltage  vd (pu)>"
  STG9/3 -> Terminator3/1
  STG9/4 -> Sum3/2, Pm9/1
  STG9/2 -> Terminator4/1
  STG9/1 -> Terminator5/1
  Bus Selector/1 -> [w9], STG9/3  "<Rotor speed  wm  (pu)>"
  Bus Selector/2 -> STG9/4, [d_theta9]  "<Rotor angle deviation  d_theta (rad)>"
  Bus Selector/3 -> Sum3/1, [Pe9]  "<Electrical power  Pe (pu)>"
  Bus Selector/4 -> Delta w PSS (Kundur) 9/1, MB-PSS9/1  "<Rotor speed deviation  dw (pu)>"
  Bus Selector/8 -> [Q9]  "<Output reactive power  Qeo (pu)>"
  Sum3/1 -> [Pa9], Delta Pa PSS 9/1  "Pm-Pe"
  Sum2/1 -> Multiport Switch1/1
  PSS model4/1 -> Sum2/2
  Delta Pa PSS 9/1 -> Multiport Switch1/5
  Delta w PSS (Kundur) 9/1 -> Multiport Switch1/4
  MB-PSS9/1 -> Multiport Switch1/3
  PSS model3/1 -> Multiport Switch1/2
  Multiport Switch1/1 -> [pss9], EXCITATION9/4
  PSS9/1 -> Sum2/1

== matlab function SCLAING_TRAINING_39/MATLAB Function ==
  data: f1 input; y output; f2 input; f3 input; f4 input; f5 input; f6 input; f7 input; f8 input; f9 input; f10 input
function y = fcn(f1,f2,f3,f4,f5,f6,f7,f8,f9,f10)
y=0.5.*(1-abs((f1-60)/0.5))+0.5.*(1-abs((f2-60)/0.5))+0.5.*(1-abs((f3-60)/0.5))+ 0.5.*(1-abs((f4-60)/0.5))+0.5.*(1-abs((f5-60)/0.5))+0.5.*(1-abs((f6-60)/0.5))+0.5.*(1-abs((f7-60)/0.5))+0.5.*(1-abs((f7-60)/0.5))+0.5.*(1-abs((f8-60)/0.5))+0.5.*(1-abs((f9-60)/0.5))+0.5.*(1-abs((f10-60)/0.5));
end




%REWARD_DEFENDER = 0.5.*(1-abs((DAF1-60)/0.5))+0.5.*(1-abs((DAF2-60)/0.5))+0.5.*(1-abs((DAF3-60)/0.5)) + 0.5.*(1-abs((DAR-4)/4)) + 0.5.*(1-abs((DATHD-10e4)/10e4));
